simulink model "PID_control"  (R2018b)
settings: Solver=VariableStepAuto  StartTime=0.0  StopTime=10  FixedStep=.001  MaxStep=.001  RelTol=1e-6  EnableMultiTasking=on
values from neighbouring files (symbols this model uses):
  armLength = 0.1    [quadcopter.m]    (also in quadcopter_control_RL.m)
  dragFactor = 0.1    [quadcopter.m]    (also in quadcopter_control_RL.m)
  iX = 0.03    [quadcopter.m]    (also in quadcopter_control_RL.m)
  iY = 0.03    [quadcopter.m]    (also in quadcopter_control_RL.m)
  iZ = 0.03    [quadcopter.m]    (also in quadcopter_control_RL.m)
  mass = 0.25    [quadcopter.m]    (also in quadcopter_control_RL.m)
  phi0 = 0.0    (= 0)    [quadcopter.m]    (also in quadcopter_control_RL.m = omega_vec_next(1))
  phiDot0 = 0.0    (= 0)    [quadcopter.m]    (also in quadcopter_control_RL.m = omega_vec_next(4))
  psi0 = 0.0    (= 0)    [quadcopter.m]    (also in quadcopter_control_RL.m = omega_vec_next(3))
  psiDot0 = 0.0    (= 0)    [quadcopter.m]    (also in quadcopter_control_RL.m = omega_vec_next(6))
  theta0 = 0.0    (= 0)    [quadcopter.m]    (also in quadcopter_control_RL.m = omega_vec_next(2))
  thetaDot0 = 0.0    (= 0)    [quadcopter.m]    (also in quadcopter_control_RL.m = omega_vec_next(5))
  thrustFactor = 0.1    [quadcopter.m]    (also in quadcopter_control_RL.m)
  x0 = 0.0    (= 0)    [quadcopter.m]    (also in quadcopter_control_RL.m = x_vec_next(1))
  xDot0 = 0.0    (= 0)    [quadcopter.m]    (also in quadcopter_control_RL.m = x_vec_next(4))
  y0 = 0.0    (= 0)    [quadcopter.m]    (also in quadcopter_control_RL.m = x_vec_next(2))
  yDot0 = 0.0    (= 0)    [quadcopter.m]    (also in quadcopter_control_RL.m = x_vec_next(5))
  z0 = 0.00000001    (= 1e-08)    [quadcopter.m]    (also in quadcopter_control_RL.m = x_vec_next(3))
  zDot0 = 0.00000001    (= 1e-08)    [quadcopter.m]    (also in quadcopter_control_RL.m = x_vec_next(6))
undefined symbols (not defined in the file or in its folder): Kd, Kp
settings Model: Creator=Andrew Petruska  LastModifiedBy=BALA BASKAR
settings OptimizationCC: LifeSpan=inf
settings DebuggingCC: SFUnexpectedBacktrackingDiag=warning  SFNoUnconditionalDefaultTransitionDiag=warning  SFExecutionAtInitializationDiag=none
settings SFSimCC: SimUseLocalCustomCode=off
settings RTWCC: RTWUseLocalCustomCode=off
settings CodeAppCC: StateflowObjectComments=on
settings GRTTargetCC: TargetLangStandard=C89/C90 (ANSI)  GeneratePreprocessorConditionals=Disable all
settings ConfigComp: CovMetricSettings=dw  CovHtmlReporting=on  CovSaveCumulativeToWorkspaceVar=on  CovSaveSingleToWorkspaceVar=on  CovExternalEMLEnable=off

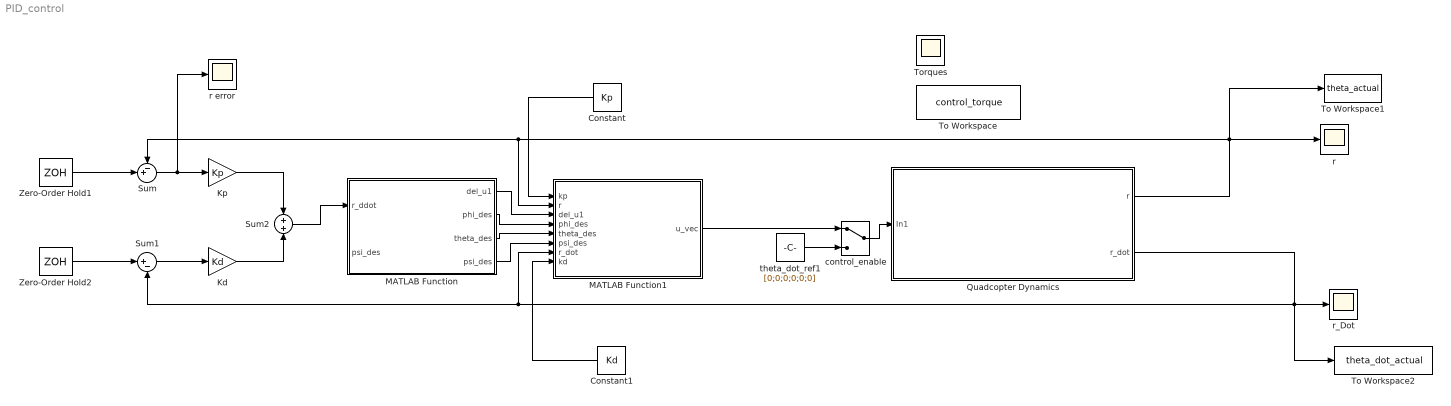
== system PID_control ==
  Constant : Constant  Value=Kp
  Constant1 : Constant  Value=Kd
  Kd : Gain  Gain=Kd
  Kp : Gain  Gain=Kp
  MATLAB Function : MATLAB Function  TreatAsAtomicUnit=on
  MATLAB Function1 : MATLAB Function  TreatAsAtomicUnit=on
  Quadcopter Dynamics : Subsystem
  Sum : Sum  Inputs=-+|
  Sum1 : Sum  Inputs=|+-
  Sum2 : Sum
  To Workspace : ToWorkspace  VariableName=control_torque  SaveFormat=Structure With Time  SampleTime=-1
  To Workspace1 : ToWorkspace  VariableName=theta_actual  SaveFormat=Structure With Time  SampleTime=-1
  To Workspace2 : ToWorkspace  VariableName=theta_dot_actual  SaveFormat=Structure With Time  SampleTime=-1
  Torques : Scope
  Zero-Order Hold1 : ZeroOrderHold  SampleTime=0.001
  Zero-Order Hold2 : ZeroOrderHold  SampleTime=0.001
  control_enable : ManualSwitch
  r : Scope
  r error : Scope
  r_Dot : Scope
  theta_dot_ref1 : Constant  Value=[0;0;0;0;0;0]
  wires:
  Quadcopter Dynamics/1(r) -> MATLAB Function1/2(r), Sum/1, r/1, To Workspace1/1
  Quadcopter Dynamics/2(r_dot) -> MATLAB Function1/7(r_dot), Sum1/2, To Workspace2/1, r_Dot/1
  Sum/1 -> r error/1, Kp/1
  Sum1/1 -> Kd/1
  Kp/1 -> Sum2/1
  Kd/1 -> Sum2/2
  Zero-Order Hold1/1 -> Sum/2
  Zero-Order Hold2/1 -> Sum1/1
  control_enable/1 -> Quadcopter Dynamics/1(In1)
  theta_dot_ref1/1 -> control_enable/2
  Sum2/1 -> MATLAB Function/1(r_ddot)
  MATLAB Function/1(del_u1) -> MATLAB Function1/3(del_u1)
  MATLAB Function/2(phi_des) -> MATLAB Function1/4(phi_des)
  MATLAB Function/3(theta_des) -> MATLAB Function1/5(theta_des)
  MATLAB Function/4(psi_des) -> MATLAB Function1/6(psi_des)
  Constant/1 -> MATLAB Function1/1(kp)
  Constant1/1 -> MATLAB Function1/8(kd)
  MATLAB Function1/1(u_vec) -> control_enable/1

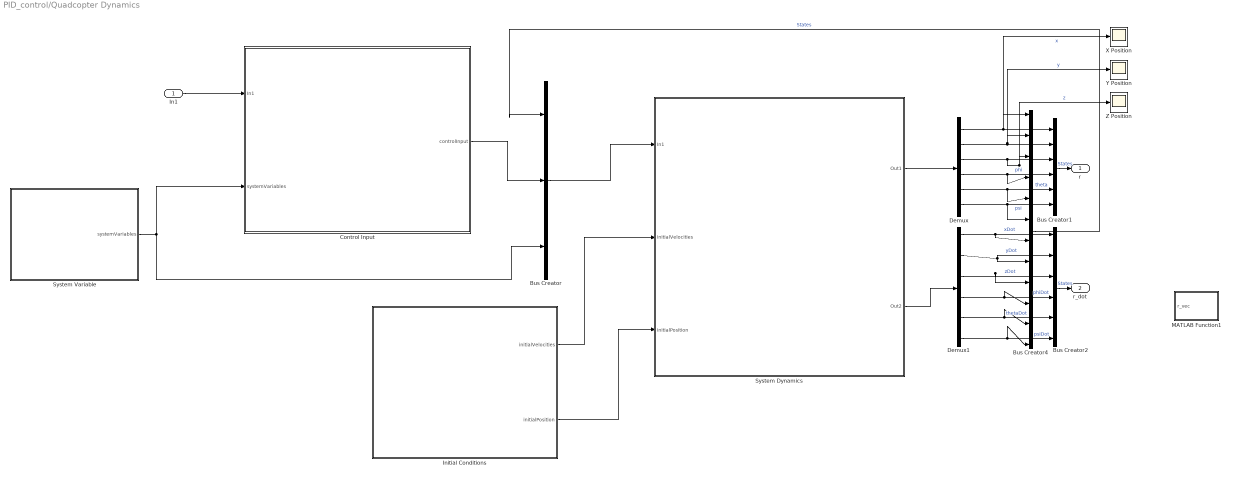
== system PID_control/Quadcopter Dynamics ==
  In1 : Inport
  Bus Creator : BusCreator  Inputs=3
  Bus Creator1 : BusCreator  Inputs=6
  Bus Creator2 : BusCreator  Inputs=6
  Bus Creator4 : BusCreator  Inputs=12
  Control Input : Subsystem
  Demux : Demux  Outputs=6
  Demux1 : Demux  Outputs=6
  Initial Conditions : Subsystem
  MATLAB Function1 : MATLAB Function  TreatAsAtomicUnit=on
  System Dynamics : Subsystem
  System Variable : Subsystem
  X Position : Scope
  Y Position : Scope
  Z Position : Scope
  r : Outport
  r_dot : Outport  Port=2
  wires:
  Initial Conditions/1(initialVelocities) -> System Dynamics/2(initialVelocities)
  Initial Conditions/2(initialPosition) -> System Dynamics/3(initialPosition)
  Bus Creator/1 -> System Dynamics/1(In1)
  Demux1/2 -> Bus Creator2/2, Bus Creator4/8  "yDot"
  Control Input/1(controlInput) -> Bus Creator/2
  System Dynamics/2(Out2) -> Demux1/1
  Demux1/3 -> Bus Creator2/3, Bus Creator4/9  "zDot"
  System Dynamics/1(Out1) -> Demux/1
  Demux/4 -> Bus Creator1/4, Bus Creator4/4  "phi"
  Demux1/5 -> Bus Creator2/5, Bus Creator4/11  "thetaDot"
  Demux/6 -> Bus Creator1/6, Bus Creator4/6  "psi"
  Demux1/4 -> Bus Creator2/4, Bus Creator4/10  "phiDot"
  Demux1/1 -> Bus Creator2/1, Bus Creator4/7  "xDot"
  Demux1/6 -> Bus Creator2/6, Bus Creator4/12  "psiDot"
  In1/1 -> Control Input/1(In1)
  Demux/1 -> X Position/1, Bus Creator1/1, Bus Creator4/1  "x"
  System Variable/1(systemVariables) -> Bus Creator/3, Control Input/2(systemVariables)
  Demux/3 -> Bus Creator1/3, Z Position/1, Bus Creator4/3  "z"
  Demux/2 -> Y Position/1, Bus Creator4/2, Bus Creator1/2  "y"
  Demux/5 -> Bus Creator1/5, Bus Creator4/5  "theta"
  Bus Creator4/1 -> Bus Creator/1  "States"
  Bus Creator1/1 -> r/1  "States"
  Bus Creator2/1 -> r_dot/1  "States"

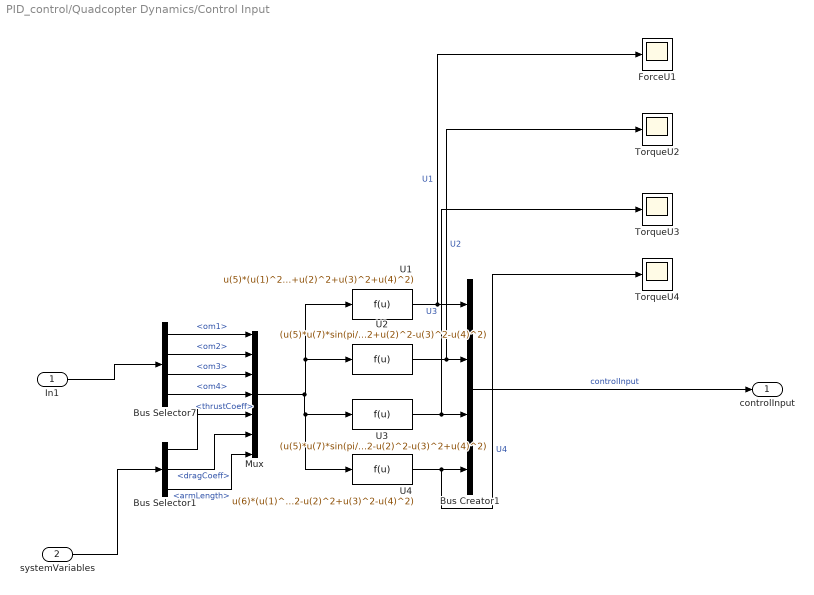
== system PID_control/Quadcopter Dynamics/Control Input ==
  In1 : Inport
  systemVariables : Inport  Port=2
  Bus Creator1 : BusCreator  Inputs=4
  Bus Selector1 : BusSelector  OutputSignals=thrustCoeff,dragCoeff,armLength
  Bus Selector7 : BusSelector  OutputSignals=om1,om2,om3,om4
  ForceU1 : Scope
  Mux : Mux  Inputs=7
  TorqueU2 : Scope
  TorqueU3 : Scope
  TorqueU4 : Scope
  U1 : Fcn  Expr=u(5)*(u(1)^2+u(2)^2+u(3)^2+u(4)^2)
  U2 : Fcn  Expr=(u(5)*u(7)*sin(pi/4))*(u(1)^2+u(2)^2-u(3)^2-u(4)^2)
  U3 : Fcn  Expr=(u(5)*u(7)*sin(pi/4))*(u(1)^2-u(2)^2-u(3)^2+u(4)^2)
  U4 : Fcn  Expr=u(6)*(u(1)^2-u(2)^2+u(3)^2-u(4)^2)
  controlInput : Outport
  wires:
  systemVariables/1 -> Bus Selector1/1
  Bus Selector7/2 -> Mux/2  "<om2>"
  Bus Selector7/4 -> Mux/4  "<om4>"
  Bus Selector7/1 -> Mux/1  "<om1>"
  U2/1 -> TorqueU2/1, Bus Creator1/2  "U2"
  Bus Selector1/2 -> Mux/6  "<dragCoeff>"
  Bus Creator1/1 -> controlInput/1  "controlInput"
  Bus Selector1/1 -> Mux/5  "<thrustCoeff>"
  U3/1 -> TorqueU3/1, Bus Creator1/3  "U3"
  Bus Selector1/3 -> Mux/7  "<armLength>"
  U4/1 -> TorqueU4/1, Bus Creator1/4  "U4"
  U1/1 -> ForceU1/1, Bus Creator1/1  "U1"
  Mux/1 -> U4/1, U3/1, U2/1, U1/1
  In1/1 -> Bus Selector7/1
  Bus Selector7/3 -> Mux/3  "<om3>"

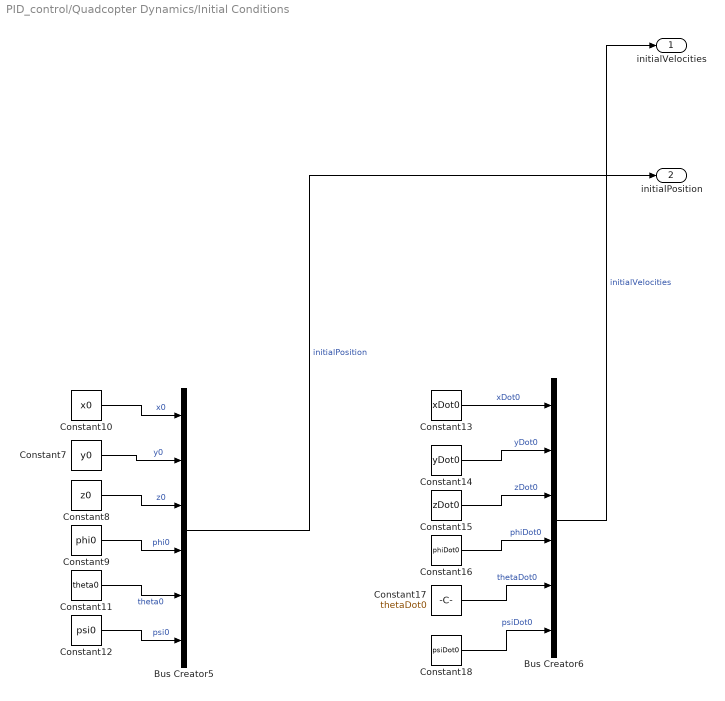
== system PID_control/Quadcopter Dynamics/Initial Conditions ==
  Bus Creator5 : BusCreator  Inputs=6
  Bus Creator6 : BusCreator  Inputs=6
  Constant10 : Constant  Value=x0
  Constant11 : Constant  Value=theta0
  Constant12 : Constant  Value=psi0
  Constant13 : Constant  Value=xDot0
  Constant14 : Constant  Value=yDot0
  Constant15 : Constant  Value=zDot0
  Constant16 : Constant  Value=phiDot0
  Constant17 : Constant  Value=thetaDot0
  Constant18 : Constant  Value=psiDot0
  Constant7 : Constant  Value=y0
  Constant8 : Constant  Value=z0
  Constant9 : Constant  Value=phi0
  initialVelocities : Outport
  initialPosition : Outport  Port=2
  wires:
  Bus Creator5/1 -> initialPosition/1  "initialPosition"
  Constant7/1 -> Bus Creator5/2  "y0"
  Bus Creator6/1 -> initialVelocities/1  "initialVelocities"
  Constant10/1 -> Bus Creator5/1  "x0"
  Constant15/1 -> Bus Creator6/3  "zDot0"
  Constant12/1 -> Bus Creator5/6  "psi0"
  Constant16/1 -> Bus Creator6/4  "phiDot0"
  Constant8/1 -> Bus Creator5/3  "z0"
  Constant11/1 -> Bus Creator5/5  "theta0"
  Constant13/1 -> Bus Creator6/1  "xDot0"
  Constant18/1 -> Bus Creator6/6  "psiDot0"
  Constant17/1 -> Bus Creator6/5  "thetaDot0"
  Constant14/1 -> Bus Creator6/2  "yDot0"
  Constant9/1 -> Bus Creator5/4  "phi0"

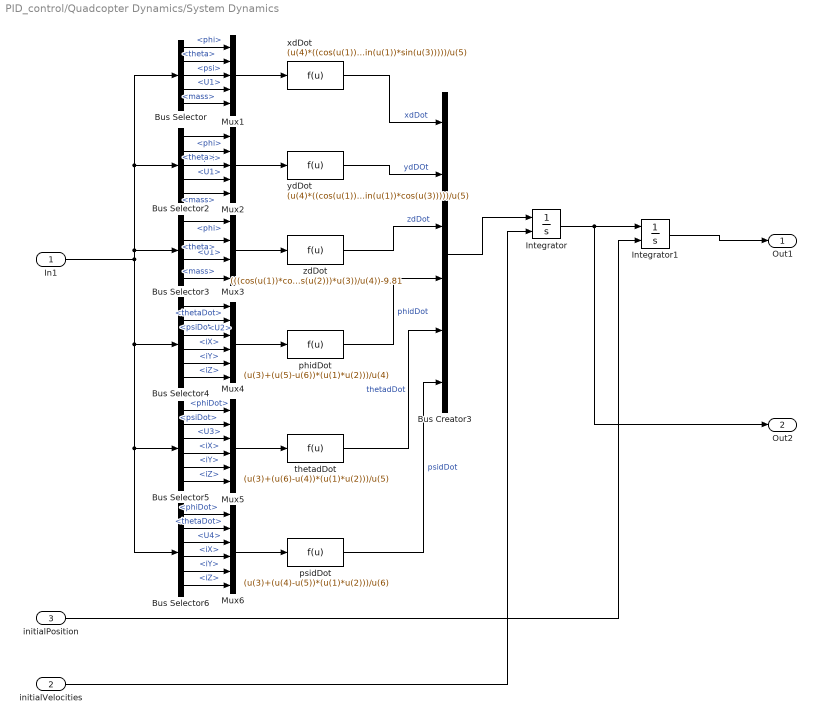
== system PID_control/Quadcopter Dynamics/System Dynamics ==
  In1 : Inport
  initialVelocities : Inport  Port=2
  initialPosition : Inport  Port=3
  Bus Creator3 : BusCreator  Inputs=6
  Bus Selector : BusSelector  OutputSignals=States.phi,States.theta,States.psi,controlInput.U1,systemVariables.mass
  Bus Selector2 : BusSelector  OutputSignals=States.phi,States.theta,States.psi,controlInput.U1,systemVariables.mass
  Bus Selector3 : BusSelector  OutputSignals=States.phi,States.theta,controlInput.U1,systemVariables.mass
  Bus Selector4 : BusSelector  OutputSignals=States.thetaDot,States.psiDot,controlInput.U2,systemVariables.iX,systemVariables.iY,systemVariables.iZ
  Bus Selector5 : BusSelector  OutputSignals=States.phiDot,States.psiDot,controlInput.U3,systemVariables.iX,systemVariables.iY,systemVariables.iZ
  Bus Selector6 : BusSelector  OutputSignals=States.phiDot,States.thetaDot,controlInput.U4,systemVariables.iX,systemVariables.iY,systemVariables.iZ
  Integrator : Integrator  InitialConditionSource=external
  Integrator1 : Integrator  InitialConditionSource=external
  Mux1 : Mux  Inputs=5
  Mux2 : Mux  Inputs=5
  Mux3 : Mux
  Mux4 : Mux  Inputs=6
  Mux5 : Mux  Inputs=6
  Mux6 : Mux  Inputs=6
  phidDot : Fcn  Expr=(u(3)+(u(5)-u(6))*(u(1)*u(2)))/u(4)
  psidDot : Fcn  Expr=(u(3)+(u(4)-u(5))*(u(1)*u(2)))/u(6)
  thetadDot : Fcn  Expr=(u(3)+(u(6)-u(4))*(u(1)*u(2)))/u(5)
  xdDot : Fcn  Expr=(u(4)*((cos(u(1))*sin(u(2))*cos(u(3)))+(sin(u(1))*sin(u(3)))))/u(5)
  ydDot : Fcn  Expr=(u(4)*((cos(u(1))*sin(u(2))*sin(u(3)))-(sin(u(1))*cos(u(3)))))/u(5)
  zdDot : Fcn  Expr=(((cos(u(1))*cos(u(2)))*u(3))/u(4))-9.81
  Out1 : Outport
  Out2 : Outport  Port=2
  wires:
  Mux1/1 -> xdDot/1
  Bus Selector3/4 -> Mux3/4  "<mass>"
  Bus Selector/2 -> Mux1/2  "<theta>"
  Bus Selector5/5 -> Mux5/5  "<iY>"
  ydDot/1 -> Bus Creator3/2  "ydDOt"
  Bus Selector/5 -> Mux1/5  "<mass>"
  Integrator1/1 -> Out1/1
  psidDot/1 -> Bus Creator3/6  "psidDot"
  Integrator/1 -> Out2/1, Integrator1/1
  Mux3/1 -> zdDot/1
  Bus Selector4/1 -> Mux4/1  "<thetaDot>"
  Bus Selector4/4 -> Mux4/4  "<iX>"
  Bus Selector6/5 -> Mux6/5  "<iY>"
  Bus Selector4/2 -> Mux4/2  "<psiDot>"
  Bus Selector5/1 -> Mux5/1  "<phiDot>"
  zdDot/1 -> Bus Creator3/3  "zdDot"
  Bus Selector6/1 -> Mux6/1  "<phiDot>"
  Bus Selector6/3 -> Mux6/3  "<U4>"
  Mux2/1 -> ydDot/1
  Bus Selector3/3 -> Mux3/3  "<U1>"
  Bus Selector6/6 -> Mux6/6  "<iZ>"
  Bus Creator3/1 -> Integrator/1
  Bus Selector2/5 -> Mux2/5  "<mass>"
  Bus Selector4/6 -> Mux4/6  "<iZ>"
  Mux4/1 -> phidDot/1
  Bus Selector/1 -> Mux1/1  "<phi>"
  Bus Selector/4 -> Mux1/4  "<U1>"
  Bus Selector5/4 -> Mux5/4  "<iX>"
  Mux6/1 -> psidDot/1
  Bus Selector/3 -> Mux1/3  "<psi>"
  initialVelocities/1 -> Integrator/2
  Bus Selector3/1 -> Mux3/1  "<phi>"
  Bus Selector3/2 -> Mux3/2  "<theta>"
  Bus Selector5/3 -> Mux5/3  "<U3>"
  In1/1 -> Bus Selector/1, Bus Selector2/1, Bus Selector3/1, Bus Selector6/1, Bus Selector5/1, Bus Selector4/1
  Bus Selector2/3 -> Mux2/3  "<psi>"
  phidDot/1 -> Bus Creator3/4  "phidDot"
  Bus Selector6/2 -> Mux6/2  "<thetaDot>"
  Bus Selector5/6 -> Mux5/6  "<iZ>"
  Bus Selector6/4 -> Mux6/4  "<iX>"
  Mux5/1 -> thetadDot/1
  Bus Selector2/1 -> Mux2/1  "<phi>"
  Bus Selector5/2 -> Mux5/2  "<psiDot>"
  thetadDot/1 -> Bus Creator3/5  "thetadDot"
  Bus Selector4/3 -> Mux4/3  "<U2>"
  Bus Selector2/4 -> Mux2/4  "<U1>"
  Bus Selector4/5 -> Mux4/5  "<iY>"
  Bus Selector2/2 -> Mux2/2  "<theta>"
  xdDot/1 -> Bus Creator3/1  "xdDot"
  initialPosition/1 -> Integrator1/2

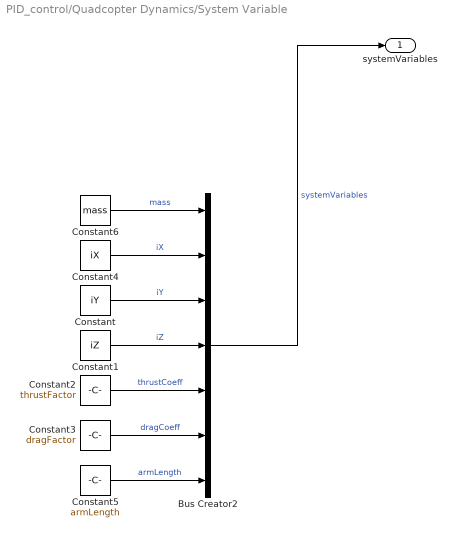
== system PID_control/Quadcopter Dynamics/System Variable ==
  Bus Creator2 : BusCreator  Inputs=7
  Constant : Constant  Value=iY
  Constant1 : Constant  Value=iZ
  Constant2 : Constant  Value=thrustFactor
  Constant3 : Constant  Value=dragFactor
  Constant4 : Constant  Value=iX
  Constant5 : Constant  Value=armLength
  Constant6 : Constant  Value=mass
  systemVariables : Outport
  wires:
  Bus Creator2/1 -> systemVariables/1  "systemVariables"
  Constant5/1 -> Bus Creator2/7  "armLength"
  Constant4/1 -> Bus Creator2/2  "iX"
  Constant3/1 -> Bus Creator2/6  "dragCoeff"
  Constant1/1 -> Bus Creator2/4  "iZ"
  Constant/1 -> Bus Creator2/3  "iY"
  Constant2/1 -> Bus Creator2/5  "thrustCoeff"
  Constant6/1 -> Bus Creator2/1  "mass"

== matlab function PID_control/Quadcopter Dynamics/MATLAB Function1 ==
  data: r_vec input
function drawDrone(r_vec)
%#codegen
coder.extrinsic('evalin');
coder.extrinsic('load');
persistent figNum axisHandel Sim_Exact points3D;

if isempty(Sim_Exact)
    Sim_Exact = evalin('base','Sim_Exact');
    a.points3D = zeros(21,3,'double');
    a = load('points3D.mat');
    points3D = zeros(21,3,'double');
    points3D = a.points3D;
end

x = r_vec(1);
y = r_vec(2);
z = r_vec(3);
phi = r_vec(4);
theta = r_vec(5);
psi = r_vec(6);

T06 = [cos(phi)*cos(theta) (cos(phi)*sin(theta)*sin(psi))-(sin(phi)*cos(psi)) (cos(phi)*sin(theta)*cos(psi))+(sin(phi)*sin(psi)) x;...
       sin(phi)*cos(theta) (sin(phi)*sin(theta)*sin(psi))+(coa(phi)*cos(psi)) (sin(phi)*sin(theta)*cos(psi))-(cos(phi)*sin(psi)) y...
       -sin(theta) (cos(theta)*sin(psi)) (sin(theta)*cos(psi)) z...
       0 0 0 1];

P1 =[ 0
    0
    0.29];
P2 = [ 0.27*cos(x)*cos(y);
    0.27*cos(y)*sin(x);
    0.29 - 0.27*sin(y)];
P3 = [ 0.27*cos(x)*cos(y) - 0.07*cos(x)*sin(y)*sin(z) + 0.07*cos(x)*cos(y)*cos(z);
    0.27*cos(y)*sin(x) - 0.07*sin(x)*sin(y)*sin(z) + 0.07*cos(y)*cos(z)*sin(x);
    0.29 - 0.07*cos(y)*sin(z) - 0.07*cos(z)*sin(y) - 0.27*sin(y)];

P4 = [ 0.27*cos(x)*cos(y) - 0.07*cos(x)*sin(y)*sin(z) + 0.07*cos(x)*cos(y)*cos(z) - 0.302*cos(x)*cos(y)*sin(z) - 0.302*cos(x)*cos(z)*sin(y);
    0.27*cos(y)*sin(x) - 0.302*cos(y)*sin(x)*sin(z) - 0.302*cos(z)*sin(x)*sin(y) - 0.07*sin(x)*sin(y)*sin(z) + 0.07*cos(y)*cos(z)*sin(x);
    0.302*sin(y)*sin(z) - 0.302*cos(y)*cos(z) - 0.07*cos(y)*sin(z) - 0.07*cos(z)*sin(y) - 0.27*sin(y) + 0.29];
P5 = [ 0.27*cos(x)*cos(y) - 0.07*cos(x)*sin(y)*sin(z) + 0.07*cos(x)*cos(y)*cos(z) - 0.302*cos(x)*cos(y)*sin(z) - 0.302*cos(x)*cos(z)*sin(y)
    0.27*cos(y)*sin(x) - 0.302*cos(y)*sin(x)*sin(z) - 0.302*cos(z)*sin(x)*sin(y) - 0.07*sin(x)*sin(y)*sin(z) + 0.07*cos(y)*cos(z)*sin(x)
    0.302*sin(y)*sin(z) - 0.302*cos(y)*cos(z) - 0.07*cos(y)*sin(z) - 0.07*cos(z)*sin(y) - 0.27*sin(y) + 0.29];

P6 =[ 0.27*cos(x)*cos(y) - 0.07*cos(x)*sin(y)*sin(z) - 0.072*sin(x)*sin(phi)*sin(theta) + 0.07*cos(x)*cos(y)*cos(z) - 0.302*cos(x)*cos(y)*sin(z) - 0.302*cos(x)*cos(z)*sin(y) - 0.072*cos(x)*cos(y)*cos(theta)*sin(z) - 0.072*cos(x)*cos(z)*cos(theta)*sin(y) - 0.072*cos(x)*cos(y)*cos(z)*cos(phi)*sin(theta) + 0.072*cos(x)*cos(phi)*sin(y)*sin(z)*sin(theta);
    0.27*cos(y)*sin(x) - 0.302*cos(y)*sin(x)*sin(z) - 0.302*cos(z)*sin(x)*sin(y) + 0.072*cos(x)*sin(phi)*sin(theta) - 0.07*sin(x)*sin(y)*sin(z) + 0.07*cos(y)*cos(z)*sin(x) - 0.072*cos(y)*cos(theta)*sin(x)*sin(z) - 0.072*cos(z)*cos(theta)*sin(x)*sin(y) - 0.072*cos(y)*cos(z)*cos(phi)*sin(x)*sin(theta) + 0.072*cos(phi)*sin(x)*sin(y)*sin(z)*sin(theta);
    0.302*sin(y)*sin(z) - 0.302*cos(y)*cos(z) - 0.07*cos(y)*sin(z) - 0.07*cos(z)*sin(y) - 0.27*sin(y) + 0.072*cos(theta)*sin(y)*sin(z) - 0.072*cos(y)*cos(z)*cos(theta) + 0.072*cos(y)*cos(phi)*sin(z)*sin(theta) + 0.072*cos(z)*cos(phi)*sin(y)*sin(theta) + 0.29];

if isempty(figNum)
    figNum = figure(1);
    hold on;
    plot3([0;P1(1);P2(1);P3(1);P4(1);P5(1);P6(1)],...
        [0;P1(2);P2(2);P3(2);P4(2);P5(2);P6(2)],...
        [0;P1(3);P2(3);P3(3);P4(3);P5(3);P6(3)],'k','linewidth',2);
    axisHandel = gca;
    plot3([P6(1);P6(1)+T06(1,1)*.1],...
        [P6(2);P6(2)+T06(2,1)*.1],...
        [P6(3);P6(3)+T06(3,1)*.1],'r','Parent',axisHandel);
    plot3([P6(1);P6(1)+T06(1,2)*.1],...
        [P6(2);P6(2)+T06(2,2)*.1],...
        [P6(3);P6(3)+T06(3,2)*.1],'g','Parent',axisHandel);
    plot3([P6(1);P6(1)+T06(1,3)*.1],...
        [P6(2);P6(2)+T06(2,3)*.1],...
        [P6(3);P6(3)+T06(3,3)*.1],'b','Parent',axisHandel);
    plot3(points3D(:,1),points3D(:,2),points3D(:,3),'m','Parent',axisHandel);
    hold off;
    axis([-.75 .75 -.75 .75 -.4 .75]);
    axisHandel = gca;
else
    plot3([0;P1(1);P2(1);P3(1);P4(1);P5(1);P6(1)],...
        [0;P1(2);P2(2);P3(2);P4(2);P5(2);P6(2)],...
        [0;P1(3);P2(3);P3(3);P4(3);P5(3);P6(3)],'k','linewidth',2,'Parent',axisHandel);
    hold on;
    plot3([P6(1);P6(1)+T06(1,1)*.1],...
        [P6(2);P6(2)+T06(2,1)*.1],...
        [P6(3);P6(3)+T06(3,1)*.1],'r','Parent',axisHandel);
    plot3([P6(1);P6(1)+T06(1,2)*.1],...
        [P6(2);P6(2)+T06(2,2)*.1],...
        [P6(3);P6(3)+T06(3,2)*.1],'g','Parent',axisHandel);
    plot3([P6(1);P6(1)+T06(1,3)*.1],...
        [P6(2);P6(2)+T06(2,3)*.1],...
        [P6(3);P6(3)+T06(3,3)*.1],'b','Parent',axisHandel);
    plot3(points3D(:,1),points3D(:,2),points3D(:,3),'m','Parent',axisHandel);
    hold off;
    axis([-.75 .75 -.75 .75 -.4 .75]);
end

== matlab function PID_control/MATLAB Function ==
  data: r_ddot input; psi_des input; del_u1 output; phi_des output; theta_des output; psi_des output
function [del_u1,phi_des,theta_des,psi_des] = POS_contol( r_ddot , psi_des )

m = 0.25;
rx_ddot = r_ddot(1);
ry_ddot = r_ddot(2);
rz_ddot = r_ddot(3);

del_u1 = m * rz_ddot;
phi_des = ((m*rx_ddot/del_u1) - (m*ry_ddot/(del_u1*tan(psi_des)))) * sin(psi_des);
theta_des = ((m*ry_ddot/del_u1) - (psi_des*cos(psi_des))) * (1/sin(psi_des));

end

== matlab function PID_control/MATLAB Function1 ==
  data: kp input; r input; del_u1 input; phi_des input; theta_des input; psi_des input; u_vec output; r_dot input; kd input
function u_vec  = Altitude_contol(kp,r,del_u1,phi_des,theta_des,psi_des,r_dot,kd)

phi_c = r(4);
theta_c = r(5);
psi_c = r(6);
phi_c_dot = r_dot(4);
theta_c_dot = r_dot(5);
psi_c_dot = r_dot(6);
del_u2 = (kp*(phi_des-phi_c))+(kd*(-1*phi_c_dot));
del_u3 = (kp*(theta_des-theta_c))+(kd*(-1*theta_c_dot));
del_u4 = (kp*(psi_des-psi_c))+(kd*(-1*psi_c_dot));

u_vec = [del_u1;del_u2;del_u3;del_u4];

end
